simulink model "camber_control"  (R2025b)
settings: Solver=ode4  StartTime=0.0  StopTime=simin.Time.data(end)  FixedStep=0.01  RelTol=1e-3
model workspace (MAT data in the model file):
  simin.Car_CFL_q0.name = 'Car.CFL.q0'
  simin.Car_CFL_q0.unit = 'm'
  simin.Car_CFL_q0.nstates = 0
  simin.Car_CFL_q0.firststate = 0
  simin.Car_CFL_q0.data = [-0.000886241672561 -0.000917774217669 -0.000942910904996 -0.000939531542826 -0.000904359389096 -0.000834426144138 -0.000731281994376 -0.000601008126978 -0.000451948289992 -0.000293444987619 -0.000134703252115 1.60676845553e-05 ... (1463 elements, 1x1463)]
  simin.Car_CFL_q2.name = 'Car.CFL.q2'
  simin.Car_CFL_q2.unit = 'm'
  simin.Car_CFL_q2.nstates = 0
  simin.Car_CFL_q2.firststate = 0
  simin.Car_CFL_q2.data = [0 3.17050847798e-07 4.58011868432e-07 -1.32496296601e-07 -7.345200288e-07 -1.22147150705e-06 -1.61682237376e-06 -1.84907457879e-06 -1.85542774034e-06 -1.63219920069e-06 -1.21697439681e-06 -6.81593121499e-07 ... (1463 elements, 1x1463)]
  simin.Car_CFL_rx.name = 'Car.CFL.rx'
  simin.Car_CFL_rx.unit = 'rad'
  simin.Car_CFL_rx.nstates = 0
  simin.Car_CFL_rx.firststate = 0
  simin.Car_CFL_rx.data = [-0.00065072166035 -0.000694006273989 -0.000704675214365 -0.000700529140886 -0.000687820604071 -0.000666201696731 -0.00063611153746 -0.000599111430347 -0.000557270133868 -0.000512964557856 -0.000468563899631 -0.000426233542385 ... (1463 elements, 1x1463)]
  simin.Car_CFL_rx_kin.name = 'Car.CFL.rx_kin'
  simin.Car_CFL_rx_kin.unit = 'rad'
  simin.Car_CFL_rx_kin.nstates = 0
  simin.Car_CFL_rx_kin.firststate = 0
  simin.Car_CFL_rx_kin.data = [-0.000256283470662 -0.000264605099801 -0.000272576377029 -0.000272559584118 -0.000263382389676 -0.000244135924731 -0.000215127511183 -0.000178044298082 -0.000135278052767 -8.95409975783e-05 -4.3526495574e-05 3.51310347924e-07 ... (1463 elements, 1x1463)]
  simin.Car_CFR_q0.name = 'Car.CFR.q0'
  simin.Car_CFR_q0.unit = 'm'
  simin.Car_CFR_q0.nstates = 0
  simin.Car_CFR_q0.firststate = 0
  simin.Car_CFR_q0.data = [-0.00088600104209 -0.000906326051336 -0.000912428018637 -0.000886603142135 -0.000829265394714 -0.000743489072192 -0.000633644813206 -0.000505556061398 -0.000365856423741 -0.000221662427066 -7.99659683253e-05 5.29072895006e-05 ... (1463 elements, 1x1463)]
  simin.Car_CFR_q2.name = 'Car.CFR.q2'
  simin.Car_CFR_q2.unit = 'm'
  simin.Car_CFR_q2.nstates = 0
  simin.Car_CFR_q2.firststate = 0
  simin.Car_CFR_q2.data = [0 3.17050847798e-07 4.58011868432e-07 -1.32496296601e-07 -7.345200288e-07 -1.22147150705e-06 -1.61682237376e-06 -1.84907457879e-06 -1.85542774034e-06 -1.63219920069e-06 -1.21697439681e-06 -6.81593121499e-07 ... (1463 elements, 1x1463)]
  simin.Car_CFR_rx.name = 'Car.CFR.rx'
  simin.Car_CFR_rx.unit = 'rad'
  simin.Car_CFR_rx.nstates = 0
  simin.Car_CFR_rx.firststate = 0
  simin.Car_CFR_rx.data = [0.000650721834973 0.000690095417667 0.000691190711223 0.000678372045513 0.000659839308355 0.000636206008494 0.000608145666774 0.000576132035349 0.000540615001228 0.000502657378092 0.000463811156806 0.000425893085776 ... (1463 elements, 1x1463)]
  simin.Car_CFR_rx_kin.name = 'Car.CFR.rx_kin'
  simin.Car_CFR_rx_kin.unit = 'rad'
  simin.Car_CFR_rx_kin.nstates = 0
  simin.Car_CFR_rx_kin.firststate = 0
  simin.Car_CFR_rx_kin.data = [0.000256283325143 0.00026183569571 0.000264437665464 0.000257808133028 0.000241926623858 0.000217718785279 0.000186409204616 0.000149691244587 0.0001094931431 6.78796204738e-05 2.68801268248e-05 -1.16706269182e-05 ... (1463 elements, 1x1463)]
  simin.Car_CRL_q0.name = 'Car.CRL.q0'
  simin.Car_CRL_q0.unit = 'm'
  simin.Car_CRL_q0.nstates = 0
  simin.Car_CRL_q0.firststate = 0
  simin.Car_CRL_q0.data = [-0.000690113112796 -0.000715000496712 -0.000763523334172 -0.000829379481729 -0.000914066913538 -0.00102130463347 -0.00115160865244 -0.00130161095876 -0.00146544119343 -0.00163598963991 -0.0018060291186 -0.00196896330453 ... (1463 elements, 1x1463)]
  simin.Car_CRL_rx.name = 'Car.CRL.rx'
  simin.Car_CRL_rx.unit = 'rad'
  simin.Car_CRL_rx.nstates = 0
  simin.Car_CRL_rx.firststate = 0
  simin.Car_CRL_rx.data = [0.0257834587246 0.0257766786963 0.0257620252669 0.0257418919355 0.0257159452885 0.0256830118597 0.0256427899003 0.0255962349474 0.0255451295525 0.0254916846752 0.0254381783307 0.0253867097199 ... (1463 elements, 1x1463)]
  simin.Car_CRL_rx_kin.name = 'Car.CRL.rx_kin'
  simin.Car_CRL_rx_kin.unit = 'rad'
  simin.Car_CRL_rx_kin.nstates = 0
  simin.Car_CRL_rx_kin.firststate = 0
  simin.Car_CRL_rx_kin.data = [0.0257834587246 0.0257766786963 0.0257620252669 0.0257418919355 0.0257159452885 0.0256830118597 0.0256427899003 0.0255962349474 0.0255451295525 0.0254916846752 0.0254381783307 0.0253867097199 ... (1463 elements, 1x1463)]
  simin.Car_CRR_q0.name = 'Car.CRR.q0'
  simin.Car_CRR_q0.unit = 'm'
  simin.Car_CRR_q0.nstates = 0
  simin.Car_CRR_q0.firststate = 0
  simin.Car_CRR_q0.data = [-0.000689887441695 -0.000704627949744 -0.000736296002287 -0.000783590483479 -0.000850609561894 -0.000944573490415 -0.00106812035665 -0.00121811509598 -0.00138789752964 -0.00156899623107 -0.00175258808304 -0.0019305361202 ... (1463 elements, 1x1463)]
  simin.Car_CRR_rx.name = 'Car.CRR.rx'
  simin.Car_CRR_rx.unit = 'rad'
  simin.Car_CRR_rx.nstates = 0
  simin.Car_CRR_rx.firststate = 0
  simin.Car_CRR_rx.data = [-0.0257834605873 -0.0257794782519 -0.0257700067014 -0.0257556829602 -0.0257353615016 -0.0257067754865 -0.0256688892841 -0.0256225410849 -0.0255697369576 -0.0255131013691 -0.0254554115236 -0.025399254635 ... (1463 elements, 1x1463)]
  simin.Car_CRR_rx_kin.name = 'Car.CRR.rx_kin'
  simin.Car_CRR_rx_kin.unit = 'rad'
  simin.Car_CRR_rx_kin.nstates = 0
  simin.Car_CRR_rx_kin.firststate = 0
  simin.Car_CRR_rx_kin.data = [-0.0257834605873 -0.0257794782519 -0.0257700067014 -0.0257556829602 -0.0257353615016 -0.0257067754865 -0.0256688892841 -0.0256225410849 -0.0255697369576 -0.0255131013691 -0.0254554115236 -0.025399254635 ... (1463 elements, 1x1463)]
  simin.Car_CamberFL.name = 'Car.CamberFL'
  simin.Car_CamberFL.unit = 'rad'
  simin.Car_CamberFL.nstates = 0
  simin.Car_CamberFL.firststate = 0
  simin.Car_CamberFL.data = [0.00065072166035 0.000694006273989 0.000704675214365 0.000700529140886 0.000687820604071 0.000666201696731 0.00063611153746 0.000599111430347 0.000557270133868 0.000512964557856 0.000468563899631 0.000426233542385 ... (1463 elements, 1x1463)]
  simin.Car_CamberFR.name = 'Car.CamberFR'
  simin.Car_CamberFR.unit = 'rad'
  simin.Car_CamberFR.nstates = 0
  simin.Car_CamberFR.firststate = 0
  simin.Car_CamberFR.data = [0.000650721834973 0.000690095417667 0.000691190711223 0.000678372045513 0.000659839308355 0.000636206008494 0.000608145666774 0.000576132035349 0.000540615001228 0.000502657378092 0.000463811156806 0.000425893085776 ... (1463 elements, 1x1463)]
  simin.Car_CamberRL.name = 'Car.CamberRL'
  simin.Car_CamberRL.unit = 'rad'
  simin.Car_CamberRL.nstates = 0
  simin.Car_CamberRL.firststate = 0
  simin.Car_CamberRL.data = [-0.0257834587246 -0.0257766786963 -0.0257620252669 -0.0257418919355 -0.0257159452885 -0.0256830118597 -0.0256427899003 -0.0255962349474 -0.0255451295525 -0.0254916846752 -0.0254381783307 -0.0253867097199 ... (1463 elements, 1x1463)]
  simin.Car_CamberRR.name = 'Car.CamberRR'
  simin.Car_CamberRR.unit = 'rad'
  simin.Car_CamberRR.nstates = 0
  simin.Car_CamberRR.firststate = 0
  simin.Car_CamberRR.data = [-0.0257834605873 -0.0257794782519 -0.0257700067014 -0.0257556829602 -0.0257353615016 -0.0257067754865 -0.0256688892841 -0.0256225410849 -0.0255697369576 -0.0255131013691 -0.0254554115236 -0.025399254635 ... (1463 elements, 1x1463)]
  simin.Car_DampFL_Frc.name = 'Car.DampFL.Frc'
  simin.Car_DampFL_Frc.unit = 'N'
  simin.Car_DampFL_Frc.nstates = 0
  simin.Car_DampFL_Frc.firststate = 0
  simin.Car_DampFL_Frc.data = [0 -9.81288814545 -4.23416090012 2.18144822121 7.28665113449 12.7316989899 17.6272563934 21.4184055328 23.8357791901 24.7871437073 24.3496685028 22.7135696411 ... (1463 elements, 1x1463)]
  simin.Car_DampFR_Frc.name = 'Car.DampFR.Frc'
  simin.Car_DampFR_Frc.unit = 'N'
  simin.Car_DampFR_Frc.nstates = 0
  simin.Car_DampFR_Frc.firststate = 0
  simin.Car_DampFR_Frc.data = [0 -5.75398349762 0.656237185001 5.79927873611 10.4937582016 14.7207098007 18.1556015015 20.6418514252 22.0629234314 22.3725852966 21.6230926514 19.9432811737 ... (1463 elements, 1x1463)]
  simin.Car_DampRL_Frc.name = 'Car.DampRL.Frc'
  simin.Car_DampRL_Frc.unit = 'N'
  simin.Car_DampRL_Frc.nstates = 0
  simin.Car_DampRL_Frc.firststate = 0
  simin.Car_DampRL_Frc.data = [0 -11.5653486252 -17.8295078278 -23.4652729034 -30.0020923615 -37.6551017761 -44.9488525391 -50.7985420227 -54.5301132202 -55.8813209534 -54.918296814 -51.9130134583 ... (1463 elements, 1x1463)]
  simin.Car_DampRR_Frc.name = 'Car.DampRR.Frc'
  simin.Car_DampRR_Frc.unit = 'N'
  simin.Car_DampRR_Frc.nstates = 0
  simin.Car_DampRR_Frc.firststate = 0
  simin.Car_DampRR_Frc.data = [0 -7.043405056 -12.0069942474 -17.3656768799 -24.582660675 -34.0090522766 -43.533782959 -51.5312919617 -57.0715255737 -59.7435531616 -59.5761260986 -56.8841400146 ... (1463 elements, 1x1463)]
  simin.Car_KinPitchCenter_L_x.name = 'Car.KinPitchCenter_L.x'
  simin.Car_KinPitchCenter_L_x.unit = 'm'
  simin.Car_KinPitchCenter_L_x.nstates = 0
  simin.Car_KinPitchCenter_L_x.firststate = 0
  simin.Car_KinPitchCenter_L_x.data = [0.504387140274 0.504779756069 0.505376279354 0.50554972887 0.505180358887 0.504185199738 0.50257641077 0.50044208765 0.497912704945 0.495144784451 0.492303609848 0.489547491074 ... (1463 elements, 1x1463)]
  simin.Car_KinPitchCenter_L_x_1.name = 'Car.KinPitchCenter_L.x_1'
  simin.Car_KinPitchCenter_L_x_1.unit = 'm'
  simin.Car_KinPitchCenter_L_x_1.nstates = 0
  simin.Car_KinPitchCenter_L_x_1.firststate = 0
  simin.Car_KinPitchCenter_L_x_1.data = [1.61338853836 1.59156286716 1.5921677351 1.59235298634 1.59199857712 1.59102213383 1.58943521976 1.58732461929 1.58481943607 1.58207523823 1.57925641537 1.57652068138 ... (1463 elements, 1x1463)]
  simin.Car_KinPitchCenter_L_y_1.name = 'Car.KinPitchCenter_L.y_1'
  simin.Car_KinPitchCenter_L_y_1.unit = 'm'
  simin.Car_KinPitchCenter_L_y_1.nstates = 0
  simin.Car_KinPitchCenter_L_y_1.firststate = 0
  simin.Car_KinPitchCenter_L_y_1.data = [0.812810838223 0.812806010246 0.812800228596 0.812796771526 0.812795162201 0.812794923782 0.812795162201 0.81279528141 0.812795162201 0.812794685364 0.812793791294 0.812792479992 ... (1463 elements, 1x1463)]
  simin.Car_KinPitchCenter_L_z.name = 'Car.KinPitchCenter_L.z'
  simin.Car_KinPitchCenter_L_z.unit = 'm'
  simin.Car_KinPitchCenter_L_z.nstates = 0
  simin.Car_KinPitchCenter_L_z.firststate = 0
  simin.Car_KinPitchCenter_L_z.data = [0.203027188778 0.203178495169 0.203405693173 0.203461542726 0.20329657197 0.202874094248 0.202196836472 0.201300188899 0.200238004327 0.199075445533 0.197881489992 0.196722269058 ... (1463 elements, 1x1463)]
  simin.Car_KinPitchCenter_L_z_1.name = 'Car.KinPitchCenter_L.z_1'
  simin.Car_KinPitchCenter_L_z_1.unit = 'm'
  simin.Car_KinPitchCenter_L_z_1.nstates = 0
  simin.Car_KinPitchCenter_L_z_1.firststate = 0
  simin.Car_KinPitchCenter_L_z_1.data = [0.181995794177 0.182137981057 0.182329982519 0.182326689363 0.182079866529 0.181553766131 0.180754169822 0.179721593857 0.178516104817 0.177209347486 0.175876200199 0.174587726593 ... (1463 elements, 1x1463)]
  simin.Car_KinPitchCenter_R_x.name = 'Car.KinPitchCenter_R.x'
  simin.Car_KinPitchCenter_R_x.unit = 'm'
  simin.Car_KinPitchCenter_R_x.nstates = 0
  simin.Car_KinPitchCenter_R_x.firststate = 0
  simin.Car_KinPitchCenter_R_x.data = [0.504397392273 0.504614770412 0.504843056202 0.504508018494 0.503591895103 0.502173602581 0.500332117081 0.498169362545 0.495796918869 0.493331938982 0.490891575813 0.488585263491 ... (1463 elements, 1x1463)]
  simin.Car_KinPitchCenter_R_x_1.name = 'Car.KinPitchCenter_R.x_1'
  simin.Car_KinPitchCenter_R_x_1.unit = 'm'
  simin.Car_KinPitchCenter_R_x_1.nstates = 0
  simin.Car_KinPitchCenter_R_x_1.firststate = 0
  simin.Car_KinPitchCenter_R_x_1.data = [1.61339890957 1.5913977623 1.59163439274 1.59131109715 1.59040987492 1.58901047707 1.58719098568 1.58505189419 1.5827037096 1.58026254177 1.57784450054 1.57555866241 ... (1463 elements, 1x1463)]
  simin.Car_KinPitchCenter_R_y_1.name = 'Car.KinPitchCenter_R.y_1'
  simin.Car_KinPitchCenter_R_y_1.unit = 'm'
  simin.Car_KinPitchCenter_R_y_1.nstates = 0
  simin.Car_KinPitchCenter_R_y_1.firststate = 0
  simin.Car_KinPitchCenter_R_y_1.data = [-0.812810778618 -0.812806904316 -0.812800586224 -0.812795877457 -0.812792778015 -0.812790811062 -0.812789857388 -0.81278949976 -0.812789618969 -0.812789857388 -0.812789916992 -0.812789678574 ... (1463 elements, 1x1463)]
  simin.Car_KinPitchCenter_R_z.name = 'Car.KinPitchCenter_R.z'
  simin.Car_KinPitchCenter_R_z.unit = 'm'
  simin.Car_KinPitchCenter_R_z.nstates = 0
  simin.Car_KinPitchCenter_R_z.firststate = 0
  simin.Car_KinPitchCenter_R_z.data = [0.203031331301 0.203111991286 0.203189015388 0.203037157655 0.202649369836 0.202055007219 0.201284185052 0.200377732515 0.199381366372 0.198343679309 0.197313711047 0.196337550879 ... (1463 elements, 1x1463)]
  simin.Car_KinPitchCenter_R_z_1.name = 'Car.KinPitchCenter_R.z_1'
  simin.Car_KinPitchCenter_R_z_1.unit = 'm'
  simin.Car_KinPitchCenter_R_z_1.nstates = 0
  simin.Car_KinPitchCenter_R_z_1.firststate = 0
  simin.Car_KinPitchCenter_R_z_1.data = [0.181999951601 0.182080060244 0.182143002748 0.181957647204 0.181512862444 0.180833622813 0.17994941771 0.178905755281 0.1777561903 0.176558405161 0.175370112062 0.174244597554 ... (1463 elements, 1x1463)]
  simin.Car_KinRollCenter_F_x_1.name = 'Car.KinRollCenter_F.x_1'
  simin.Car_KinRollCenter_F_x_1.unit = 'm'
  simin.Car_KinRollCenter_F_x_1.nstates = 0
  simin.Car_KinRollCenter_F_x_1.firststate = 0
  simin.Car_KinRollCenter_F_x_1.data = [4.08391618729 4.06163883209 4.06161642075 4.06162166595 4.06163978577 4.06166744232 4.06170082092 4.06173610687 4.06177186966 4.06180620193 4.06183862686 4.06186819077 ... (1463 elements, 1x1463)]
  simin.Car_KinRollCenter_F_y.name = 'Car.KinRollCenter_F.y'
  simin.Car_KinRollCenter_F_y.unit = 'm'
  simin.Car_KinRollCenter_F_y.nstates = 0
  simin.Car_KinRollCenter_F_y.firststate = 0
  simin.Car_KinRollCenter_F_y.data = [2.19647540689e-06 3.56523960363e-05 7.55673390813e-05 0.000106820938527 0.000134184898343 0.000148567210999 0.000144712990732 0.0001275613904 0.00010418335296 8.01177375251e-05 5.88769071328e-05 4.18086456193e-05 ... (1463 elements, 1x1463)]
  simin.Car_KinRollCenter_F_y_1.name = 'Car.KinRollCenter_F.y_1'
  simin.Car_KinRollCenter_F_y_1.unit = 'm'
  simin.Car_KinRollCenter_F_y_1.nstates = 0
  simin.Car_KinRollCenter_F_y_1.firststate = 0
  simin.Car_KinRollCenter_F_y_1.data = [2.197422873e-06 3.47701279679e-05 7.32885309844e-05 0.00010392274271 0.000131741107907 0.000147430080688 0.000145377780427 0.000130054890178 0.000108112217276 8.48645504448e-05 6.37928387732e-05 4.63463838969e-05 ... (1463 elements, 1x1463)]
  simin.Car_KinRollCenter_F_z.name = 'Car.KinRollCenter_F.z'
  simin.Car_KinRollCenter_F_z.unit = 'm'
  simin.Car_KinRollCenter_F_z.nstates = 0
  simin.Car_KinRollCenter_F_z.firststate = 0
  simin.Car_KinRollCenter_F_z.data = [0.106545142829 0.106592237949 0.106617286801 0.106594793499 0.106523685157 0.106404274702 0.106240786612 0.106042675674 0.105822078884 0.10559219867 0.105365715921 0.105153590441 ... (1463 elements, 1x1463)]
  simin.Car_KinRollCenter_F_z_1.name = 'Car.KinRollCenter_F.z_1'
  simin.Car_KinRollCenter_F_z_1.unit = 'm'
  simin.Car_KinRollCenter_F_z_1.nstates = 0
  simin.Car_KinRollCenter_F_z_1.firststate = 0
  simin.Car_KinRollCenter_F_z_1.data = [0.0853210985661 0.0853669047356 0.0853967368603 0.0853973701596 0.0853716507554 0.0853234827518 0.0852594971657 0.0851862132549 0.085108757019 0.0850312933326 0.0849572569132 0.084889434278 ... (1463 elements, 1x1463)]
  simin.Car_KinRollCenter_R_x_1.name = 'Car.KinRollCenter_R.x_1'
  simin.Car_KinRollCenter_R_x_1.unit = 'm'
  simin.Car_KinRollCenter_R_x_1.nstates = 0
  simin.Car_KinRollCenter_R_x_1.firststate = 0
  simin.Car_KinRollCenter_R_x_1.data = [1.10899782181 1.08677971363 1.086789608 1.08680522442 1.08682656288 1.08685445786 1.08688807487 1.08692574501 1.08696520329 1.08700454235 1.08704209328 1.08707654476 ... (1463 elements, 1x1463)]
  simin.Car_KinRollCenter_R_y.name = 'Car.KinRollCenter_R.y'
  simin.Car_KinRollCenter_R_y.unit = 'm'
  simin.Car_KinRollCenter_R_y.nstates = 0
  simin.Car_KinRollCenter_R_y.firststate = 0
  simin.Car_KinRollCenter_R_y.data = [-6.46729887421e-08 -3.83480837627e-05 -0.000136810704134 -0.000256856146734 -0.000373983406462 -0.000463141332148 -0.000506969634444 -0.000502845156007 -0.000458209746284 -0.000384902086807 -0.000295471952995 -0.000200780807063 ... (1463 elements, 1x1463)]
  simin.Car_KinRollCenter_R_y_1.name = 'Car.KinRollCenter_R.y_1'
  simin.Car_KinRollCenter_R_y_1.unit = 'm'
  simin.Car_KinRollCenter_R_y_1.nstates = 0
  simin.Car_KinRollCenter_R_y_1.firststate = 0
  simin.Car_KinRollCenter_R_y_1.data = [-6.4395990762e-08 -3.90070999856e-05 -0.000137729584821 -0.000257737672655 -0.000374666880816 -0.000463525211671 -0.000507078249939 -0.000502789800521 -0.000458104419522 -0.000384825660149 -0.000295459700283 -0.000200833237614 ... (1463 elements, 1x1463)]
  simin.Car_KinRollCenter_R_z.name = 'Car.KinRollCenter_R.z'
  simin.Car_KinRollCenter_R_z.unit = 'm'
  simin.Car_KinRollCenter_R_z.nstates = 0
  simin.Car_KinRollCenter_R_z.firststate = 0
  simin.Car_KinRollCenter_R_z.data = [0.0665587410331 0.0665603280067 0.0665664896369 0.0665797069669 0.0666007995605 0.0666302889585 0.0666679218411 0.066712141037 0.0667605251074 0.0668103843927 0.0668591484427 0.0669047087431 ... (1463 elements, 1x1463)]
  simin.Car_KinRollCenter_R_z_1.name = 'Car.KinRollCenter_R.z_1'
  simin.Car_KinRollCenter_R_z_1.unit = 'm'
  simin.Car_KinRollCenter_R_z_1.nstates = 0
  simin.Car_KinRollCenter_R_z_1.firststate = 0
  simin.Car_KinRollCenter_R_z_1.data = [0.0455666817725 0.0455627404153 0.0455382838845 0.0454909913242 0.0454191938043 0.0453207679093 0.0451966449618 0.045051984489 0.0448944978416 0.0447327457368 0.0445747412741 0.0444271117449 ... (1463 elements, 1x1463)]
  simin.Car_Pitch.name = 'Car.Pitch'
  simin.Car_Pitch.unit = 'rad'
  simin.Car_Pitch.nstates = 0
  simin.Car_Pitch.firststate = 0
  simin.Car_Pitch.data = [-7.79904221417e-05 -7.52850028221e-05 -6.04346387263e-05 -2.8753947845e-05 2.16319476749e-05 9.28526642383e-05 0.000184566975804 0.000292904151138 0.000411792017985 0.000534345686901 0.000654050207231 0.000765468284953 ... (1463 elements, 1x1463)]
  simin.Car_PitchAcc.name = 'Car.PitchAcc'
  simin.Car_PitchAcc.unit = 'rad/s^2'
  simin.Car_PitchAcc.nstates = 0
  simin.Car_PitchAcc.firststate = 0
  simin.Car_PitchAcc.data = [-0.00852889381349 0.121664367616 0.168117746711 0.183017984033 0.209351181984 0.21022169292 0.173254534602 0.112930946052 0.0432575829327 -0.0232661813498 -0.0791773051023 -0.121358901262 ... (1463 elements, 1x1463)]
  simin.Car_PitchVel.name = 'Car.PitchVel'
  simin.Car_PitchVel.unit = 'rad/s'
  simin.Car_PitchVel.nstates = 0
  simin.Car_PitchVel.firststate = 0
  simin.Car_PitchVel.data = [-8.52889388625e-06 0.000697757466696 0.00219570402987 0.00398324336857 0.00594714889303 0.00808134768158 0.0100052533671 0.0114194955677 0.0121677452698 0.0122277392074 0.0116769401357 0.0106417741627 ... (1463 elements, 1x1463)]
  simin.Car_Roll.name = 'Car.Roll'
  simin.Car_Roll.unit = 'rad'
  simin.Car_Roll.nstates = 0
  simin.Car_Roll.firststate = 0
  simin.Car_Roll.data = [1.43921411677e-07 7.44030921851e-06 2.12926825043e-05 3.72147878807e-05 5.20691428392e-05 6.2607730797e-05 6.69595683576e-05 6.51424124953e-05 5.83028668188e-05 4.80521921418e-05 3.60137019015e-05 2.35477309616e-05 ... (1463 elements, 1x1463)]
  simin.Car_RollAcc.name = 'Car.RollAcc'
  simin.Car_RollAcc.unit = 'rad/s^2'
  simin.Car_RollAcc.nstates = 0
  simin.Car_RollAcc.firststate = 0
  simin.Car_RollAcc.data = [0.135388016701 0.0696013346314 0.0224885232747 -0.00593412248418 -0.0415635295212 -0.0628033578396 -0.0632719546556 -0.0520820505917 -0.0358180776238 -0.0191673096269 -0.00512819783762 0.00499975075945 ... (1463 elements, 1x1463)]
  simin.Car_RollVel.name = 'Car.RollVel'
  simin.Car_RollVel.unit = 'rad/s'
  simin.Car_RollVel.nstates = 0
  simin.Car_RollVel.firststate = 0
  simin.Car_RollVel.data = [0.00013538802159 0.00111896626186 0.00153417419642 0.00159765814897 0.0013381280005 0.00079064280726 0.000145676502143 -0.000432054774137 -0.000865363399498 -0.0011307480745 -0.00124280131422 -0.00123484688811 ... (1463 elements, 1x1463)]
  simin.Car_SlipAngleFL.name = 'Car.SlipAngleFL'
  simin.Car_SlipAngleFL.unit = 'rad'
  simin.Car_SlipAngleFL.nstates = 0
  simin.Car_SlipAngleFL.firststate = 0
  simin.Car_SlipAngleFL.data = [0.00274525093846 0.00254377769306 0.00250400300138 0.00250612595119 0.00251825316809 0.00252945558168 0.00253392313607 0.00253175012767 0.00252496404573 0.00251550134271 0.00250486657023 0.00249378592707 ... (1463 elements, 1x1463)]
  simin.Car_SlipAngleFR.name = 'Car.SlipAngleFR'
  simin.Car_SlipAngleFR.unit = 'rad'
  simin.Car_SlipAngleFR.nstates = 0
  simin.Car_SlipAngleFR.firststate = 0
  simin.Car_SlipAngleFR.data = [-0.00274524791166 -0.00249069393612 -0.00243572099134 -0.00245000561699 -0.00248308014125 -0.00252318824641 -0.00255724578165 -0.00257763452828 -0.0025836781133 -0.00257754488848 -0.00256266235374 -0.00254241097718 ... (1463 elements, 1x1463)]
  simin.Car_SlipAngleRL.name = 'Car.SlipAngleRL'
  simin.Car_SlipAngleRL.unit = 'rad'
  simin.Car_SlipAngleRL.nstates = 0
  simin.Car_SlipAngleRL.firststate = 0
  simin.Car_SlipAngleRL.data = [0.0019979889039 0.00200552283786 0.00200556102209 0.0019967420958 0.00197870703414 0.00195213453844 0.00192474899814 0.00190290645696 0.00188955641352 0.00188533868641 0.00188929610886 0.00189968128689 ... (1463 elements, 1x1463)]
  simin.Car_SlipAngleRR.name = 'Car.SlipAngleRR'
  simin.Car_SlipAngleRR.unit = 'rad'
  simin.Car_SlipAngleRR.nstates = 0
  simin.Car_SlipAngleRR.firststate = 0
  simin.Car_SlipAngleRR.data = [-0.0019979889039 -0.00195941887796 -0.00194127042778 -0.00193320622202 -0.00193066848442 -0.00193212321028 -0.00193584605586 -0.0019398429431 -0.00194356124848 -0.00194715335965 -0.0019510933198 -0.00195587123744 ... (1463 elements, 1x1463)]
  simin.Car_SpringFL_Frc.name = 'Car.SpringFL.Frc'
  simin.Car_SpringFL_Frc.unit = 'N'
  simin.Car_SpringFL_Frc.nstates = 0
  simin.Car_SpringFL_Frc.firststate = 0
  simin.Car_SpringFL_Frc.data = [3699.37353516 3698.52832031 3697.72119141 3697.73144531 3698.66699219 3700.61889648 3703.55834961 3707.31665039 3711.65356445 3716.29614258 3720.97192383 3725.43603516 ... (1463 elements, 1x1463)]
  simin.Car_SpringFR_Frc.name = 'Car.SpringFR.Frc'
  simin.Car_SpringFR_Frc.unit = 'N'
  simin.Car_SpringFR_Frc.nstates = 0
  simin.Car_SpringFR_Frc.firststate = 0
  simin.Car_SpringFR_Frc.data = [3699.37548828 3698.8190918 3698.55834961 3699.21948242 3700.81567383 3703.25683594 3706.4206543 3710.13916016 3714.21948242 3718.453125 3722.63378906 3726.57275391 ... (1463 elements, 1x1463)]
  simin.Car_SpringRL_Frc.name = 'Car.SpringRL.Frc'
  simin.Car_SpringRL_Frc.unit = 'N'
  simin.Car_SpringRL_Frc.nstates = 0
  simin.Car_SpringRL_Frc.firststate = 0
  simin.Car_SpringRL_Frc.data = [3300.99462891 3300.13110352 3298.2644043 3295.69970703 3292.39428711 3288.19897461 3283.07519531 3277.14453125 3270.63427734 3263.82592773 3257.01000977 3250.45336914 ... (1463 elements, 1x1463)]
  simin.Car_SpringRR_Frc.name = 'Car.SpringRR.Frc'
  simin.Car_SpringRR_Frc.unit = 'N'
  simin.Car_SpringRR_Frc.nstates = 0
  simin.Car_SpringRR_Frc.firststate = 0
  simin.Car_SpringRR_Frc.data = [3300.99658203 3300.48950195 3299.28295898 3297.45825195 3294.86938477 3291.2277832 3286.40185547 3280.49755859 3273.77075195 3266.55615234 3259.20703125 3252.05322266 ... (1463 elements, 1x1463)]
  simin.Car_StabiFL_Frc.name = 'Car.StabiFL.Frc'
  simin.Car_StabiFL_Frc.unit = 'N'
  simin.Car_StabiFL_Frc.nstates = 0
  simin.Car_StabiFL_Frc.firststate = 0
  simin.Car_StabiFL_Frc.data = [7.82602728577e-06 0.128220692277 0.370446920395 0.658734798431 0.951356232166 1.16804897785 1.26733720303 1.24952304363 1.13573861122 0.954649269581 0.735302388668 0.502714037895 ... (1463 elements, 1x1463)]
  simin.Car_StabiFR_Frc.name = 'Car.StabiFR.Frc'
  simin.Car_StabiFR_Frc.unit = 'N'
  simin.Car_StabiFR_Frc.nstates = 0
  simin.Car_StabiFR_Frc.firststate = 0
  simin.Car_StabiFR_Frc.data = [-7.82602728577e-06 -0.128220692277 -0.370446920395 -0.658734798431 -0.951356232166 -1.16804897785 -1.26733720303 -1.24952304363 -1.13573861122 -0.954649269581 -0.735302388668 -0.502714037895 ... (1463 elements, 1x1463)]
  simin.Car_StabiRL_Frc.name = 'Car.StabiRL.Frc'
  simin.Car_StabiRL_Frc.unit = 'N'
  simin.Car_StabiRL_Frc.nstates = 0
  simin.Car_StabiRL_Frc.firststate = 0
  simin.Car_StabiRL_Frc.data = [9.64909268077e-05 0.133757278323 0.381350755692 0.65880048275 0.927548348904 1.13517642021 1.24684000015 1.25672841072 1.17556905746 1.02315247059 0.823290109634 0.599329173565 ... (1463 elements, 1x1463)]
  simin.Car_StabiRR_Frc.name = 'Car.StabiRR.Frc'
  simin.Car_StabiRR_Frc.unit = 'N'
  simin.Car_StabiRR_Frc.nstates = 0
  simin.Car_StabiRR_Frc.firststate = 0
  simin.Car_StabiRR_Frc.data = [-9.64909268077e-05 -0.133757278323 -0.381350755692 -0.65880048275 -0.927548348904 -1.13517642021 -1.24684000015 -1.25672841072 -1.17556905746 -1.02315247059 -0.823290109634 -0.599329173565 ... (1463 elements, 1x1463)]
  simin.Car_SteerAngleFL.name = 'Car.SteerAngleFL'
  simin.Car_SteerAngleFL.unit = 'rad'
  simin.Car_SteerAngleFL.nstates = 0
  simin.Car_SteerAngleFL.firststate = 0
  simin.Car_SteerAngleFL.data = [-0.00274520018138 -0.00253772852011 -0.00247604819015 -0.00246139639057 -0.0024629808031 -0.00246950471774 -0.00247323769145 -0.00247170752846 -0.00246601528488 -0.00245808321051 -0.00244981329888 -0.00244237133302 ... (1463 elements, 1x1463)]
  simin.Car_SteerAngleFR.name = 'Car.SteerAngleFR'
  simin.Car_SteerAngleFR.unit = 'rad'
  simin.Car_SteerAngleFR.nstates = 0
  simin.Car_SteerAngleFR.firststate = 0
  simin.Car_SteerAngleFR.data = [0.00274519715458 0.00253069470637 0.00247041904368 0.00246500223875 0.00247227377258 0.00248133391142 0.00248558609746 0.00248261680827 0.00247403862886 0.00246242946014 0.00245020748116 0.00243902229704 ... (1463 elements, 1x1463)]
  simin.Car_SteerAngleRL.name = 'Car.SteerAngleRL'
  simin.Car_SteerAngleRL.unit = 'rad'
  simin.Car_SteerAngleRL.nstates = 0
  simin.Car_SteerAngleRL.firststate = 0
  simin.Car_SteerAngleRL.data = [-0.00200000009499 -0.00200000009499 -0.00200000009499 -0.00200000009499 -0.00200000009499 -0.00200000009499 -0.00200000009499 -0.00200000009499 -0.00200000009499 -0.00200000009499 -0.00200000009499 -0.00200000009499 ... (1463 elements, 1x1463)]
  simin.Car_SteerAngleRR.name = 'Car.SteerAngleRR'
  simin.Car_SteerAngleRR.unit = 'rad'
  simin.Car_SteerAngleRR.nstates = 0
  simin.Car_SteerAngleRR.firststate = 0
  simin.Car_SteerAngleRR.data = [0.00200000009499 0.00200000009499 0.00200000009499 0.00200000009499 0.00200000009499 0.00200000009499 0.00200000009499 0.00200000009499 0.00200000009499 0.00200000009499 0.00200000009499 0.00200000009499 ... (1463 elements, 1x1463)]
  simin.Car_ax.name = 'Car.ax'
  simin.Car_ax.unit = 'm/s^2'
  simin.Car_ax.nstates = 0
  simin.Car_ax.firststate = 0
  simin.Car_ax.data = [-0.457714706659 -0.534651875496 -0.662543535233 -0.741658329964 -0.843395709991 -0.914263963699 -0.900133371353 -0.828636705875 -0.726416051388 -0.619259238243 -0.523548901081 -0.446759223938 ... (1463 elements, 1x1463)]
  simin.Car_ay.name = 'Car.ay'
  simin.Car_ay.unit = 'm/s^2'
  simin.Car_ay.nstates = 0
  simin.Car_ay.firststate = 0
  simin.Car_ay.data = [0.0283882785589 -0.00948819238693 -0.00888870749623 -0.00742548424751 -0.00492731528357 -0.000478249799926 0.00372694525868 0.00648484425619 0.00785560160875 0.00800772663206 0.00728780031204 0.0060185464099 ... (1463 elements, 1x1463)]
  simin.Car_az.name = 'Car.az'
  simin.Car_az.unit = 'm/s^2'
  simin.Car_az.nstates = 0
  simin.Car_az.firststate = 0
  simin.Car_az.data = [1.57921946049 0.0678590387106 0.0510664507747 0.0390611626208 0.0383150093257 0.0183799322695 0.000791482860222 -0.012433427386 -0.0206380598247 -0.0241861790419 -0.0245063286275 -0.0227154940367 ... (1463 elements, 1x1463)]
  simin.Car_tx.name = 'Car.tx'
  simin.Car_tx.unit = 'm'
  simin.Car_tx.nstates = 0
  simin.Car_tx.firststate = 0
  simin.Car_tx.data = [2.61795282364 2.84016108513 3.0623190403 3.28441166878 3.50642991066 3.72836446762 3.9502081871 4.1719622612 4.39363288879 4.61523103714 4.83676624298 5.05824899673 ... (1463 elements, 1x1463)]
  simin.Car_ty.name = 'Car.ty'
  simin.Car_ty.unit = 'm'
  simin.Car_ty.nstates = 0
  simin.Car_ty.firststate = 0
  simin.Car_ty.data = [-5.15416775926e-09 -2.92536327606e-07 -1.17966783364e-06 -2.73618593383e-06 -4.8594688451e-06 -7.28459053789e-06 -9.68172389548e-06 -1.17478948596e-05 -1.32604300234e-05 -1.40986567203e-05 -1.423861886e-05 -1.37315673783e-05 ... (1463 elements, 1x1463)]
  simin.Car_tz.name = 'Car.tz'
  simin.Car_tz.unit = 'm'
  simin.Car_tz.nstates = 0
  simin.Car_tz.firststate = 0
  simin.Car_tz.data = [0.625109732151 0.62511330843 0.625121891499 0.625134706497 0.625151395798 0.62517118454 0.625193357468 0.625216901302 0.625240981579 0.625264883041 0.625288069248 0.625310182571 ... (1463 elements, 1x1463)]
  simin.Car_v.name = 'Car.v'
  simin.Car_v.unit = 'm/s'
  simin.Car_v.nstates = 0
  simin.Car_v.firststate = 0
  simin.Car_v.data = [22.2222213745 22.2189311981 22.2130565643 22.2060241699 22.1982498169 22.1894168854 22.1802597046 22.1715068817 22.1636257172 22.1568069458 22.1510238647 22.1461238861 ... (1463 elements, 1x1463)]
  simin.Steer_L_q.name = 'Steer.L.q'
  simin.Steer_L_q.unit = 'm'
  simin.Steer_L_q.nstates = 0
  simin.Steer_L_q.firststate = 0
  simin.Steer_L_q.data = [0 3.17050847798e-07 4.58011868432e-07 -1.32496296601e-07 -7.345200288e-07 -1.22147150705e-06 -1.61682237376e-06 -1.84907457879e-06 -1.85542774034e-06 -1.63219920069e-06 -1.21697439681e-06 -6.81593121499e-07 ... (1463 elements, 1x1463)]
  simin.Steer_R_q.name = 'Steer.R.q'
  simin.Steer_R_q.unit = 'm'
  simin.Steer_R_q.nstates = 0
  simin.Steer_R_q.firststate = 0
  simin.Steer_R_q.data = [0 3.17050847798e-07 4.58011868432e-07 -1.32496296601e-07 -7.345200288e-07 -1.22147150705e-06 -1.61682237376e-06 -1.84907457879e-06 -1.85542774034e-06 -1.63219920069e-06 -1.21697439681e-06 -6.81593121499e-07 ... (1463 elements, 1x1463)]
  simin.Steer_RL_q.name = 'Steer.RL.q'
  simin.Steer_RL_q.unit = 'm'
  simin.Steer_RL_q.nstates = 0
  simin.Steer_RL_q.firststate = 0
  simin.Steer_RL_q.data = [0 0 0 0 0 0 0 0 0 0 0 0 ... (1463 elements, 1x1463)]
  simin.Steer_RR_q.name = 'Steer.RR.q'
  simin.Steer_RR_q.unit = 'm'
  simin.Steer_RR_q.nstates = 0
  simin.Steer_RR_q.firststate = 0
  simin.Steer_RR_q.data = [0 0 0 0 0 0 0 0 0 0 0 0 ... (1463 elements, 1x1463)]
  simin.Time.name = 'Time'
  simin.Time.unit = 's'
  simin.Time.nstates = 0
  simin.Time.firststate = 0
  simin.Time.data = [0 0.01 0.02 0.03 0.04 0.05 0.06 0.07 0.08 0.09 0.1 0.11 ... (1463 elements, 1x1463)]
undefined symbols (not defined in the file): camberMapFL, compression, compression_FL, compression_FR, DiscIntNeverNeededParam, distance_to_pitch_center_front, steer, steering_rack_displacement_FL, steering_rack_displacement_FR, track_width_front, track_width_rear, wheelbase
settings Model: DataDictionary=vehicleData.sldd  EnableAccessToBaseWorkspace=off  Creator=marce  LastModifiedBy=marce

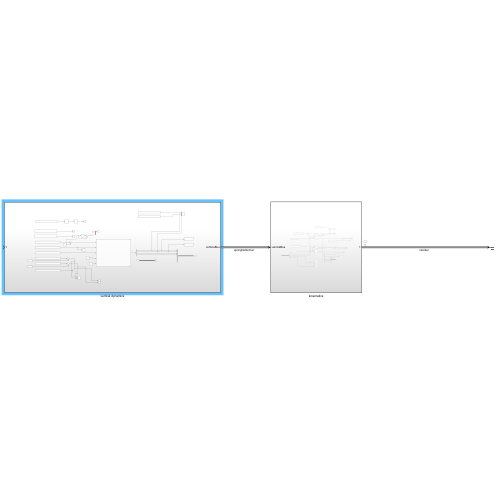
[thumbnail: Simulink's stored preview of the top-level diagram]
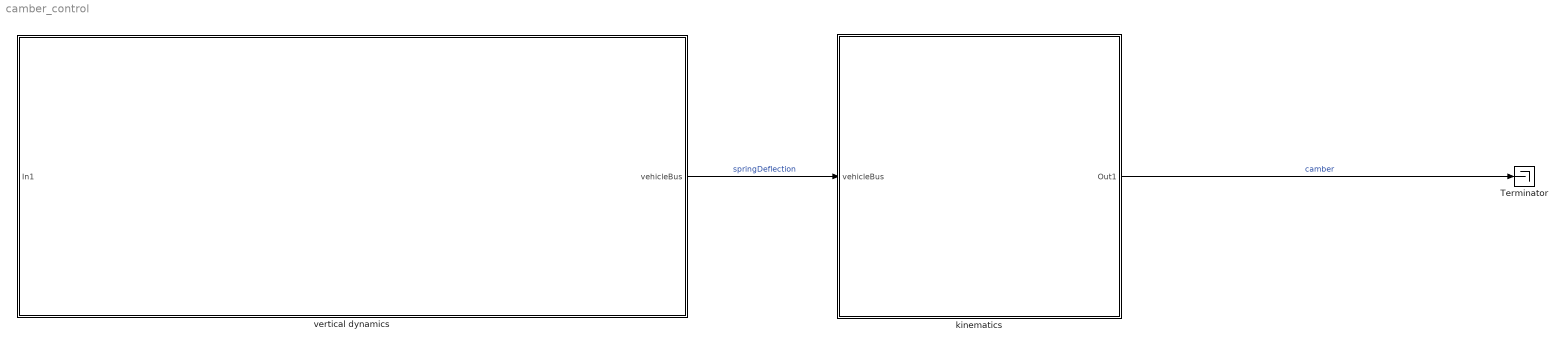
== system camber_control ==
  Terminator : Terminator
  kinematics : Subsystem
  vertical dynamics : Subsystem
  wires:
  vertical dynamics/1(vehicleBus) -> kinematics/1(vehicleBus)  "springDeflection"
  kinematics/1(Out1) -> Terminator/1  "camber"

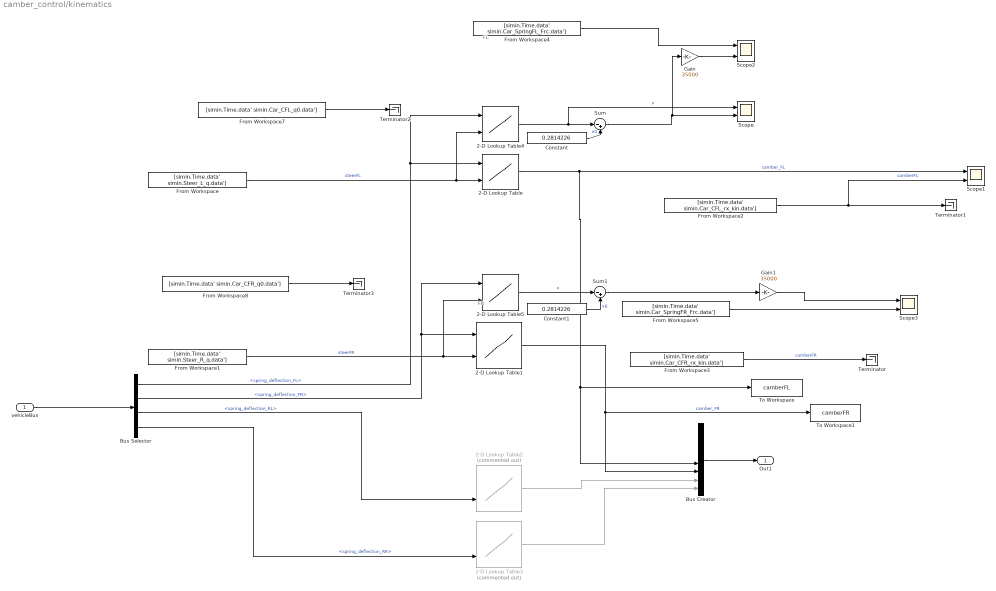
== system camber_control/kinematics ==
  note: FL
  note: FR
  vehicleBus : Inport  OutDataTypeStr=Bus: camberControlBus
  2-D Lookup Table : Lookup_n-D  BreakpointsForDimension1=compression_FL  BreakpointsForDimension2=steering_rack_displacement_FL  Table=camber_map_FL'  InterpMethod=Linear Lagrange  InternalRulePriority=Speed  RndMeth=Simplest
      settings: InputPortMap=u0,u1
  2-D Lookup Table1 : Lookup_n-D  BreakpointsForDimension1=compression_FR  BreakpointsForDimension2=steering_rack_displacement_FR  Table=camber_map_FR'  InterpMethod=Linear Lagrange  InternalRulePriority=Speed  RndMeth=Simplest
      settings: InputPortMap=u0,u1
  2-D Lookup Table2 : Lookup_n-D  Commented=on  BreakpointsForDimension1=steer.*10^3'  BreakpointsForDimension2=compression.*10^3  Table=camberMapFL  InternalRulePriority=Speed  RndMeth=Simplest
      settings: InputPortMap=u0,u1
  2-D Lookup Table3 : Lookup_n-D  Commented=on  BreakpointsForDimension1=steer.*10^3'  BreakpointsForDimension2=compression.*10^3  Table=camberMapFL  InternalRulePriority=Speed  RndMeth=Simplest
      settings: InputPortMap=u0,u1
  2-D Lookup Table4 : Lookup_n-D  BreakpointsForDimension1=compression_FL  BreakpointsForDimension2=steering_rack_displacement_FL  Table=spring_map_FL'  InternalRulePriority=Speed  RndMeth=Simplest
      settings: InputPortMap=u0,u1
  2-D Lookup Table5 : Lookup_n-D  BreakpointsForDimension1=compression_FR  BreakpointsForDimension2=steering_rack_displacement_FR  Table=spring_map_FR'  InternalRulePriority=Speed  RndMeth=Simplest
      settings: InputPortMap=u0,u1
  Bus Creator : BusCreator  Inputs=8  OutDataTypeStr=Bus: camberControlBus
      settings: InheritFromInputs=off
  Bus Selector : BusSelector  OutputSignals=spring_deflection_FL,spring_deflection_FR,spring_deflection_RL,spring_deflection_RR
  Constant : Constant  Value=0.2814226
  Constant1 : Constant  Value=0.2814226
  From Workspace : FromWorkspace  VariableName=[simin.Time.data' simin.Steer_L_q.data']
  From Workspace1 : FromWorkspace  VariableName=[simin.Time.data' simin.Steer_R_q.data']
  From Workspace2 : FromWorkspace  VariableName=[simin.Time.data' simin.Car_CFL_rx_kin.data']
  From Workspace3 : FromWorkspace  VariableName=[simin.Time.data' simin.Car_CFR_rx_kin.data']
  From Workspace4 : FromWorkspace  VariableName=[simin.Time.data' simin.Car_SpringFL_Frc.data']
  From Workspace5 : FromWorkspace  VariableName=[simin.Time.data' simin.Car_SpringFR_Frc.data']
  From Workspace7 : FromWorkspace  VariableName=[simin.Time.data' simin.Car_CFL_q0.data']
  From Workspace8 : FromWorkspace  VariableName=[simin.Time.data' simin.Car_CFR_q0.data']
  Gain : Gain  Gain=35000
  Gain1 : Gain  Gain=35000
  Scope{,1..3} (4 alike) : Scope  NumInputPorts=2
      Scope settings: ActiveDisplayYMinimum=-1  ActiveDisplayYMaximum=1
      Scope1 settings: ActiveDisplayYMinimum=-1  ActiveDisplayYMaximum=1  DataLoggingVariableName=ScopeData5
      Scope2 settings: ActiveDisplayYMinimum=2814.6166700708645  ActiveDisplayYMaximum=5704.3374513167519  DataLoggingVariableName=ScopeData2
      Scope3 settings: ActiveDisplayYMinimum=3121.4952529789343  ActiveDisplayYMaximum=5432.2058225856736  DataLoggingVariableName=ScopeData6
  Sum : Sum  Inputs=|-+
  Sum1 : Sum  Inputs=|-+
  Terminator{,1..3} (4 alike) : Terminator
  To Workspace : ToWorkspace  VariableName=camberFL  SampleTime=0.01
      settings: Save2DSignal=2-D array (concatenate along first dimension)
  To Workspace1 : ToWorkspace  VariableName=camberFR  SampleTime=0.01
      settings: Save2DSignal=2-D array (concatenate along first dimension)
  Out1 : Outport  OutDataTypeStr=Bus: camberControlBus
  wires:
  2-D Lookup Table/1 -> Bus Creator/5, To Workspace/1, Scope1/1  "camber_FL"
  2-D Lookup Table1/1 -> Bus Creator/6, To Workspace1/1  "camber_FR"
  vehicleBus/1 -> Bus Selector/1
  Bus Selector/1 -> 2-D Lookup Table4/1, 2-D Lookup Table/1  "<spring_deflection_FL>"
  Bus Selector/2 -> 2-D Lookup Table1/1, 2-D Lookup Table5/1  "<spring_deflection_FR>"
  Bus Selector/3 -> 2-D Lookup Table2/2  "<spring_deflection_RL>"
  Bus Selector/4 -> 2-D Lookup Table3/2  "<spring_deflection_RR>"
  Bus Creator/1 -> Out1/1
  2-D Lookup Table2/1 -> Bus Creator/7
  2-D Lookup Table3/1 -> Bus Creator/8
  From Workspace/1 -> 2-D Lookup Table4/2, 2-D Lookup Table/2  "steerFL"
  From Workspace3/1 -> Terminator/1  "camberFR"
  From Workspace2/1 -> Terminator1/1, Scope1/2  "camberFL"
  From Workspace8/1 -> Terminator3/1
  From Workspace1/1 -> 2-D Lookup Table5/2, 2-D Lookup Table1/2  "steerFR"
  2-D Lookup Table4/1 -> Scope/1, Sum/1  "x"
  From Workspace4/1 -> Scope2/1
  Gain/1 -> Scope2/2
  From Workspace7/1 -> Terminator2/1
  Constant/1 -> Sum/2  "x0"
  Sum/1 -> Gain/1, Scope/2
  2-D Lookup Table5/1 -> Sum1/1  "x"
  Constant1/1 -> Sum1/2  "x0"
  Sum1/1 -> Gain1/1
  Gain1/1 -> Scope3/1
  From Workspace5/1 -> Scope3/2

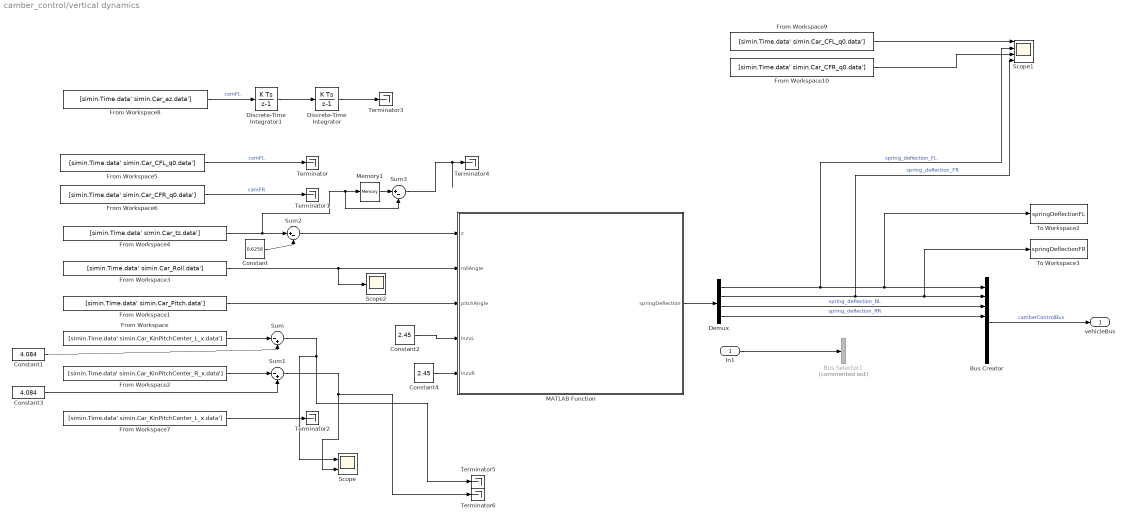
== system camber_control/vertical dynamics ==
  In1 : Inport  OutDataTypeStr=Bus: camberControlBus
  Bus Creator : BusCreator  Inputs=8  OutDataTypeStr=Bus: camberControlBus
  Bus Selector1 : BusSelector  Commented=on  OutputSignals=signal1,signal2
  Constant : Constant  Value=0.6258
  Constant1 : Constant  Value=4.084
  Constant2 : Constant  Value=2.45
  Constant3 : Constant  Value=4.084
  Constant4 : Constant  Value=2.45
  Demux : Demux
  Discrete-Time Integrator : DiscreteIntegrator  InitialCondition=0.626  SampleTime=-1  ICPrevOutput=DiscIntNeverNeededParam  ICPrevScaledInput=DiscIntNeverNeededParam
  Discrete-Time Integrator1 : DiscreteIntegrator  SampleTime=-1  ICPrevOutput=DiscIntNeverNeededParam  ICPrevScaledInput=DiscIntNeverNeededParam
  From Workspace : FromWorkspace  VariableName=[simin.Time.data' simin.Car_KinPitchCenter_L_x.data']
  From Workspace1 : FromWorkspace  VariableName=[simin.Time.data' simin.Car_Pitch.data']
  From Workspace10 : FromWorkspace  VariableName=[simin.Time.data' simin.Car_CFR_q0.data']
  From Workspace2 : FromWorkspace  VariableName=[simin.Time.data' simin.Car_KinPitchCenter_R_x.data']
  From Workspace3 : FromWorkspace  VariableName=[simin.Time.data' simin.Car_Roll.data']
  From Workspace4 : FromWorkspace  VariableName=[simin.Time.data' simin.Car_tz.data']
  From Workspace5 : FromWorkspace  VariableName=[simin.Time.data' simin.Car_CFL_q0.data']
  From Workspace6 : FromWorkspace  VariableName=[simin.Time.data' simin.Car_CFR_q0.data']
  From Workspace7 : FromWorkspace  VariableName=[simin.Time.data' simin.Car_KinPitchCenter_L_x.data']
  From Workspace8 : FromWorkspace  VariableName=[simin.Time.data' simin.Car_az.data']  OutDataTypeStr=double
  From Workspace9 : FromWorkspace  VariableName=[simin.Time.data' simin.Car_CFL_q0.data']
  MATLAB Function : MATLAB Function  TreatAsAtomicUnit=on
  Memory1 : Memory  InitialCondition=simin.Car_tz.data(1)'
  Scope : Scope  NumInputPorts=2
      settings: ActiveDisplayYMinimum=0.69571051859860145  ActiveDisplayYMaximum=18.182643094300822
  Scope1 : Scope  NumInputPorts=4
      settings: ActiveDisplayYMinimum=-0.020516756926986866  ActiveDisplayYMaximum=0.057429901014320925  DataLoggingVariableName=ScopeData3
  Scope2 : Scope
      settings: ActiveDisplayYMinimum=-1  ActiveDisplayYMaximum=1  DataLoggingVariableName=ScopeData4
  Sum : Sum  Inputs=|-+
  Sum1 : Sum  Inputs=|-+
  Sum2 : Sum  Inputs=|+-
  Sum3 : Sum  Inputs=|+-
  Terminator{,1..6} (7 alike) : Terminator
  To Workspace2 : ToWorkspace  VariableName=springDeflectionFL  SampleTime=0.01
      settings: Save2DSignal=2-D array (concatenate along first dimension)
  To Workspace3 : ToWorkspace  VariableName=springDeflectionFR  SampleTime=0.01
      settings: Save2DSignal=2-D array (concatenate along first dimension)
  vehicleBus : Outport
  wires:
  MATLAB Function/1(springDeflection) -> Demux/1
  Demux/1 -> Scope1/2, To Workspace2/1, Bus Creator/1  "spring_deflection_FL"
  Demux/2 -> Bus Creator/2, To Workspace3/1, Scope1/4  "spring_deflection_FR"
  Bus Creator/1 -> vehicleBus/1  "camberControlBus"
  Demux/3 -> Bus Creator/3  "spring_deflection_RL"
  Demux/4 -> Bus Creator/4  "spring_deflection_RR"
  In1/1 -> Bus Selector1/1
  From Workspace/1 -> Sum/1
  Constant1/1 -> Sum/2
  From Workspace2/1 -> Sum1/1
  Constant3/1 -> Sum1/2
  From Workspace5/1 -> Terminator/1  "comFL"
  Sum2/1 -> MATLAB Function/1(z)
  From Workspace6/1 -> Terminator1/1  "camFR"
  Sum/1 -> Terminator5/1, Scope/1
  From Workspace8/1 -> Discrete-Time Integrator1/1  "comFL"
  Discrete-Time Integrator1/1 -> Discrete-Time Integrator/1
  Discrete-Time Integrator/1 -> Terminator3/1
  From Workspace7/1 -> Terminator2/1
  Sum1/1 -> Terminator6/1, Scope/2
  From Workspace1/1 -> MATLAB Function/3(pitchAngle)
  From Workspace3/1 -> Scope2/1, MATLAB Function/2(rollAngle)
  From Workspace9/1 -> Scope1/1
  From Workspace10/1 -> Scope1/3
  Memory1/1 -> Sum3/1
  From Workspace4/1 -> Memory1/1, Sum3/2, Sum2/1
  Sum3/1 -> Terminator4/1
  Constant/1 -> Sum2/2
  Constant2/1 -> MATLAB Function/4(lnzvL)
  Constant4/1 -> MATLAB Function/5(lnzvR)

== matlab function camber_control/vertical dynamics/MATLAB Function ==
  data: z input double; rollAngle input; springDeflection output; pitchAngle input; wheelbase parameter; distance_to_pitch_center_front parameter; track_width_rear parameter; track_width_front parameter; lnzvL input; lnzvR input
function springDeflection = wheel_elevation(z, rollAngle, pitchAngle, ...
    wheelbase, distance_to_pitch_center_front, track_width_rear, track_width_front, lnzvL, lnzvR)

l = wheelbase;
sv = track_width_front;
sh = track_width_rear;
%lnzv = distance_to_pitch_center_front;

z1 = z - sin(rollAngle) * (sv/2) + sin(pitchAngle) * lnzvL;     % vorne links
z2 = z + sin(rollAngle) * (sv/2) + sin(pitchAngle) * lnzvR;     % vorne rechts
z3 = z - sin(rollAngle) * (sh/2) - sin(pitchAngle) * (l-lnzvL); % hinten links
z4 = z + sin(rollAngle) * (sh/2) - sin(pitchAngle) * (l-lnzvR); % hinten rechts

springDeflection = [z1, z2, z3, z4];
